simulink model "T_TEM_112"  (R2015a)
settings: Solver=ode3  StartTime=0.0  StopTime=5  FixedStep=1  RelTol=1e-3
values from neighbouring files (symbols this model uses):
  I = 4.1    [Untitled.m]
  T_c1 = 288    [Untitled.m]
  T_c2 = 288    [Untitled.m]
  T_h1 = 396    [Untitled.m]
  T_h2 = 381    [Untitled.m]
libraries: LU_TEG x2
settings Model: Creator=lansong7  LastModifiedBy=lansong7

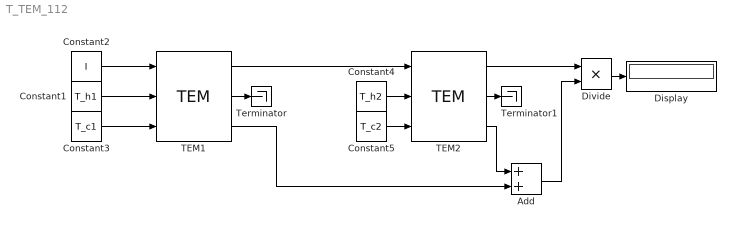
== system T_TEM_112 ==
  Add : Sum
  Constant1 : Constant  Value=T_h1
  Constant2 : Constant  Value=I
  Constant3 : Constant  Value=T_c1
  Constant4 : Constant  Value=T_h2
  Constant5 : Constant  Value=T_c2
  Display : Display
  Divide : Product  Inputs=**
  TEM1 : LU_TEG/TEM  l=l  l_cw=l_cw  f=f  a=a  n=n  Tune_tr=Tune_tr  Tune_er=Tune_er  ct1=ct1  ct2=ct2
  TEM2 : LU_TEG/TEM  l=l  l_cw=l_cw  f=f  a=a  n=n  Tune_tr=Tune_tr  Tune_er=Tune_er  ct1=ct1  ct2=ct2
  Terminator : Terminator
  Terminator1 : Terminator
  wires:
  Constant1/1 -> TEM1/2
  Constant3/1 -> TEM1/3
  Constant2/1 -> TEM1/1
  TEM1/1 -> TEM2/1
  TEM1/2 -> Terminator/1
  TEM2/2 -> Terminator1/1
  TEM2/1 -> Divide/1
  Constant4/1 -> TEM2/2
  Constant5/1 -> TEM2/3
  TEM2/3 -> Add/1
  TEM1/3 -> Add/2
  Divide/1 -> Display/1
  Add/1 -> Divide/2
